simulink model "DCmotor2"  (Simulink 8.0)
settings: Solver=ode45  StartTime=0  StopTime=2000  FixedStep=0.005  RelTol=1e-3
settings Model: Creator=Tran Minh Luan  LastModifiedBy=Tran Minh Luan

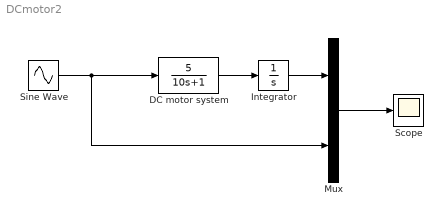
== system DCmotor2 ==
  DC motor system : TransferFcn  Numerator=[5]  Denominator=[10 1]
  Integrator : Integrator
  Mux : Mux  Inputs=2
  Scope : Scope
      settings: TickLabels=on
  Sine Wave : Sin  Amplitude=10  Frequency=0.01  SampleTime=0
  wires:
  Mux/1 -> Scope/1
  DC motor system/1 -> Integrator/1
  Integrator/1 -> Mux/1
  Sine Wave/1 -> Mux/2, DC motor system/1
